simulink model "sampleModel180"  (R2021b)
settings: Solver=VariableStepAuto  StartTime=0.0  StopTime=10.0  RelTol=1e-3
undefined symbols (not defined in the file or in its folder): DiscIntNeverNeededParam, Newton, Raphson
libraries: simulink x11, slpidlib x4
settings Model: Creator=user  LastModifiedBy=user

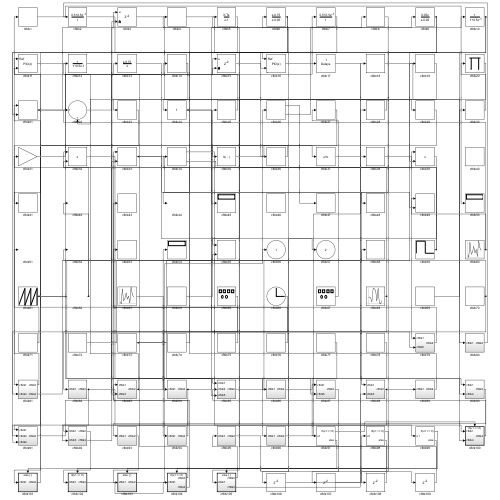
[thumbnail: Simulink's stored preview of the top-level diagram]
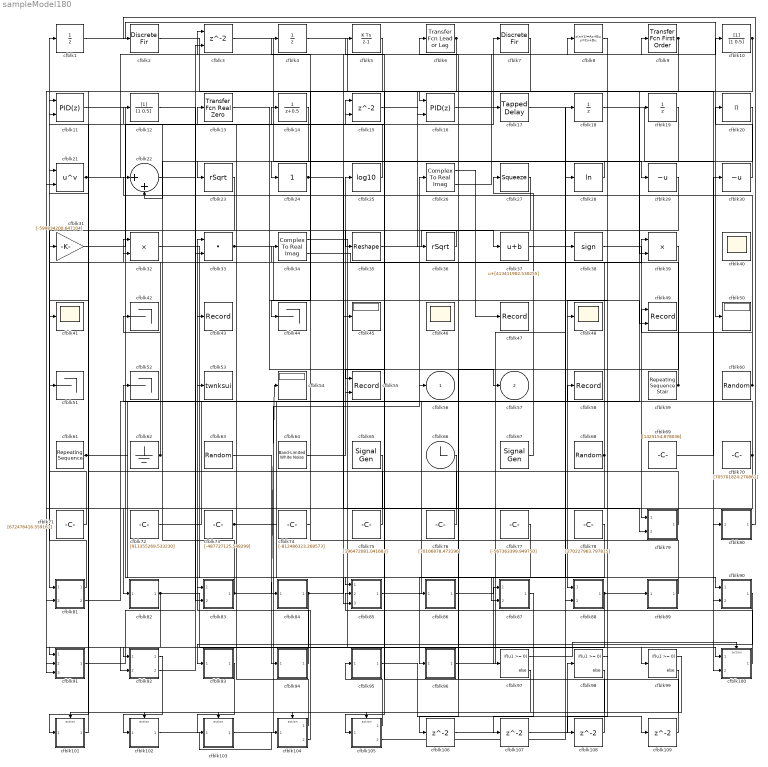
== system sampleModel180 ==
  cfblk{1,4,18..19} (4 alike) : UnitDelay  HasFrameUpgradeWarning=on
  cfblk10 : DiscreteFilter  SampleTime=1
  cfblk100 : Subsystem  TreatAsAtomicUnit=on
  cfblk101 : Subsystem  TreatAsAtomicUnit=on
  cfblk102 : Subsystem  TreatAsAtomicUnit=on
  cfblk103 : Subsystem  TreatAsAtomicUnit=on
  cfblk104 : Subsystem  TreatAsAtomicUnit=on
  cfblk105 : Subsystem  TreatAsAtomicUnit=on
  cfblk{106..109} (4 alike) : Delay  SampleTime=1
  cfblk11 : slpidlib/PID Controller (2DOF)  Controller=PID  Form=Parallel  TimeDomain=Discrete-time  UseExternalTs=off  SampleTime=1  IntegratorMethod=Forward Euler  FilterMethod=Forward Euler  ControllerParametersSource=internal  P=1  I=1  D=0  UseFilter=on  N=100  b=1  c=1  TunerSelectOption=Transfer Function Based (PID Tuner App)  InitialConditionSource=internal  InitialConditionForIntegrator=0  InitialConditionForFilter=0  DifferentiatorICPrevScaledInput=0  ExternalReset=none  TrackingMode=off  Kt=1  LimitOutput=off  SatLimitsSource=internal  UpperSaturationLimit=inf  LowerSaturationLimit=-inf  LinearizeAsGain=off  AntiWindupMode=none  Kb=1  POutMin=[]  POutMax=[]  IOutMin=[]  IOutMax=[]  DOutMin=[]  DOutMax=[]  NOutMin=[]  NOutMax=[]  bOutMin=[]  bOutMax=[]  cOutMin=[]  cOutMax=[]  SumOutMin=[]  SumOutMax=[]  SaturationOutMin=[]  SaturationOutMax=[]  PParamMin=[]  PParamMax=[]  IParamMin=[]  IParamMax=[]  DParamMin=[]  DParamMax=[]  NParamMin=[]  NParamMax=[]  bParamMin=[]  bParamMax=[]  cParamMin=[]  cParamMax=[]  KbParamMin=[]  KbParamMax=[]  KtParamMin=[]  KtParamMax=[]  KbOutMin=[]  KbOutMax=[]  KtOutMin=[]  KtOutMax=[]  IntegratorOutMin=[]  IntegratorOutMax=[]  FilterOutMin=[]  FilterOutMax=[]  SumI1OutMin=[]  SumI1OutMax=[]  SumI2OutMin=[]  SumI2OutMax=[]  SumI3OutMin=[]  SumI3OutMax=[]  SumI4OutMin=[]  SumI4OutMax=[]  SumDOutMin=[]  SumDOutMax=[]  Sum1OutMin=[]  Sum1OutMax=[]  Sum2OutMin=[]  Sum2OutMax=[]  Sum3OutMin=[]  Sum3OutMax=[]  DifferentiatorOutMin=[]  DifferentiatorOutMax=[]  FilterDiffOutCoefMin=[]  FilterDiffOutCoefMax=[]  ReciprocalOutMin=[]  ReciprocalOutMax=[]  SumDenOutMin=[]  SumDenOutMax=[]  SumNumOutMin=[]  SumNumOutMax=[]  DivideOutMin=[]  DivideOutMax=[]  UdiffTsProdOutMin=[]  UdiffTsProdOutMax=[]  NTsProdOutMin=[]  NTsProdOutMax=[]  UintegralTsProdOutMin=[]  UintegralTsProdOutMax=[]  UngainTsProdOutMin=[]  UngainTsProdOutMax=[]  IntegratorContinuousStateAttributes=''  IntegratorStateMustResolveToSignalObject=off  IntegratorRTWStateStorageClass=Auto  FilterContinuousStateAttributes=''  FilterStateMustResolveToSignalObject=off  FilterRTWStateStorageClass=Auto  ParallelPVariant=InternalParameters  IdealPVariant=Disabled  IVariant=InternalParameters  DVariant=InternalParameters  bVariant=InternalParameters  cVariant=InternalParameters  IntegratorVariant=Discrete  SatVariant=Disabled  AWVariant=Passthrough  PCopyVariant=Disabled  TRVariant=Disabled  FdbkBlocksVariant=Forward  IdealPFdbkVariant=Disabled  SatFdbkVariant=Disabled  DerivativeFilterVariant=ForwardEulerFilter  NVariant=InternalParameters  NCopyVariant=Disabled  FilterICVariant=InternalICsFilter  IntegratorICVariant=InternalICs  ExternalResetVariant=Disabled  TRSumVariant=Passthrough  SumFdbkVariant=Disabled  SumVariant=Sum_PID  TsampFilterVariant=InternalTs  TsampNgainVariant=Passthrough  TsampIntegralVariant=Passthrough  ExternalSaturationOutDataTypeStr=Inherit: Same as second input
      settings: SourceProductBaseCode=SL
  cfblk12 : DiscreteFilter  SampleTime=1
  cfblk13 : simulink/Discrete/Transfer Fcn Real Zero  ZeroZ=0.75  ICPrevInput=0.0  DoSatur=off
      settings: SourceProductBaseCode=SL
  cfblk14 : DiscreteTransferFcn  SampleTime=1
  cfblk15 : Delay  ShowEnablePort=on  SampleTime=1
      settings: InputPortMap=u0,e6
  cfblk16 : slpidlib/PID Controller (2DOF)  Controller=PID  Form=Parallel  TimeDomain=Discrete-time  UseExternalTs=off  SampleTime=1  IntegratorMethod=Forward Euler  FilterMethod=Forward Euler  ControllerParametersSource=internal  P=1  I=1  D=0  UseFilter=on  N=100  b=1  c=1  TunerSelectOption=Transfer Function Based (PID Tuner App)  InitialConditionSource=internal  InitialConditionForIntegrator=0  InitialConditionForFilter=0  DifferentiatorICPrevScaledInput=0  ExternalReset=none  TrackingMode=off  Kt=1  LimitOutput=off  SatLimitsSource=internal  UpperSaturationLimit=inf  LowerSaturationLimit=-inf  LinearizeAsGain=off  AntiWindupMode=none  Kb=1  POutMin=[]  POutMax=[]  IOutMin=[]  IOutMax=[]  DOutMin=[]  DOutMax=[]  NOutMin=[]  NOutMax=[]  bOutMin=[]  bOutMax=[]  cOutMin=[]  cOutMax=[]  SumOutMin=[]  SumOutMax=[]  SaturationOutMin=[]  SaturationOutMax=[]  PParamMin=[]  PParamMax=[]  IParamMin=[]  IParamMax=[]  DParamMin=[]  DParamMax=[]  NParamMin=[]  NParamMax=[]  bParamMin=[]  bParamMax=[]  cParamMin=[]  cParamMax=[]  KbParamMin=[]  KbParamMax=[]  KtParamMin=[]  KtParamMax=[]  KbOutMin=[]  KbOutMax=[]  KtOutMin=[]  KtOutMax=[]  IntegratorOutMin=[]  IntegratorOutMax=[]  FilterOutMin=[]  FilterOutMax=[]  SumI1OutMin=[]  SumI1OutMax=[]  SumI2OutMin=[]  SumI2OutMax=[]  SumI3OutMin=[]  SumI3OutMax=[]  SumI4OutMin=[]  SumI4OutMax=[]  SumDOutMin=[]  SumDOutMax=[]  Sum1OutMin=[]  Sum1OutMax=[]  Sum2OutMin=[]  Sum2OutMax=[]  Sum3OutMin=[]  Sum3OutMax=[]  DifferentiatorOutMin=[]  DifferentiatorOutMax=[]  FilterDiffOutCoefMin=[]  FilterDiffOutCoefMax=[]  ReciprocalOutMin=[]  ReciprocalOutMax=[]  SumDenOutMin=[]  SumDenOutMax=[]  SumNumOutMin=[]  SumNumOutMax=[]  DivideOutMin=[]  DivideOutMax=[]  UdiffTsProdOutMin=[]  UdiffTsProdOutMax=[]  NTsProdOutMin=[]  NTsProdOutMax=[]  UintegralTsProdOutMin=[]  UintegralTsProdOutMax=[]  UngainTsProdOutMin=[]  UngainTsProdOutMax=[]  IntegratorContinuousStateAttributes=''  IntegratorStateMustResolveToSignalObject=off  IntegratorRTWStateStorageClass=Auto  FilterContinuousStateAttributes=''  FilterStateMustResolveToSignalObject=off  FilterRTWStateStorageClass=Auto  ParallelPVariant=InternalParameters  IdealPVariant=Disabled  IVariant=InternalParameters  DVariant=InternalParameters  bVariant=InternalParameters  cVariant=InternalParameters  IntegratorVariant=Discrete  SatVariant=Disabled  AWVariant=Passthrough  PCopyVariant=Disabled  TRVariant=Disabled  FdbkBlocksVariant=Forward  IdealPFdbkVariant=Disabled  SatFdbkVariant=Disabled  DerivativeFilterVariant=ForwardEulerFilter  NVariant=InternalParameters  NCopyVariant=Disabled  FilterICVariant=InternalICsFilter  IntegratorICVariant=InternalICs  ExternalResetVariant=Disabled  TRSumVariant=Passthrough  SumFdbkVariant=Disabled  SumVariant=Sum_PID  TsampFilterVariant=InternalTs  TsampNgainVariant=Passthrough  TsampIntegralVariant=Passthrough  ExternalSaturationOutDataTypeStr=Inherit: Same as second input
      settings: SourceProductBaseCode=SL
  cfblk17 : simulink/Discrete/Tapped Delay  vinit=0.0  samptime=-1  NumDelays=1  DelayOrder=Oldest  includeCurrent=off
  cfblk2 : DiscreteFir  SampleTime=1
  cfblk20 : Product  Inputs=*
  cfblk21 : Math  Operator=pow  SaturateOnIntegerOverflow=on
  cfblk22 : Sum  Inputs=|++
  cfblk23 : Sqrt  Operator=rSqrt  AlgorithmType=Newton-Raphson  SaturateOnIntegerOverflow=on
  cfblk24 : simulink/Math Operations/Slider Gain  gain=1  low=0  high=2
  cfblk25 : Math  Operator=log10  SaturateOnIntegerOverflow=on
  cfblk26 : ComplexToRealImag
  cfblk27 : Squeeze
  cfblk28 : Math  Operator=log  SaturateOnIntegerOverflow=on
  cfblk29 : UnaryMinus
  cfblk3 : Delay  ShowEnablePort=on  SampleTime=1
      settings: InputPortMap=u0,e6
  cfblk30 : UnaryMinus
  cfblk31 : Gain  Gain=[-599834200.647104]
  cfblk32 : Product
  cfblk33 : DotProduct  InputSameDT=on  OutDataTypeStr=Inherit: Inherit via internal rule
  cfblk34 : ComplexToRealImag
  cfblk35 : Reshape
  cfblk36 : Sqrt  Operator=rSqrt  AlgorithmType=Newton-Raphson  SaturateOnIntegerOverflow=on
  cfblk37 : Bias  Bias=[413411902.530255]
  cfblk38 : Signum
  cfblk39 : Product
  cfblk{40..41,46,48} (4 alike) : Scope
      cfblk40 settings: Floating=on
      cfblk46 settings: Floating=on
  cfblk{42,44,51..52} (4 alike) : Terminator
  cfblk43 : Record  FileSettingsInternal="{\"entries\":[{\"content\":{\"excelSettings\":{\"content\":{},\"type\":\"Streamout.ExcelSettings\"}},\"type\":\"Streamout.FileSettingStorage\",\"uuid\":\"86445610-928e-4e35-9d69-0b2c780a0add\"}],\"packageUris\":[\"http://schema.mathworks.com/mf0/streamout_blocks/R2020a\"],\"version\":\"1.0\"}"  SignalsInternal="{\"entries\":[{\"content\":{\"signals\":[{\"content\":{\"blockPath\":[\"sampleModel180/cfblk43\"],\"channel\":[],\"dimensions\":[1],\"domain\":\"sampleModel180/cfblk43\",\"lineColor\":\"#4dbeee\",\"plots\":[1],\"port\":1,\"sid\":[\"\"],\"signalID\":6746,\"signalName\":\"cfblk79\"},\"type\":\"RecordBlkView.Signal\",\"uuid\":\"ec482149-7623-4eb4-899c-afc25818783d\"}]},\"type\":\"RecordBlkView.InputSignals\",\"uuid\":\"a47f1734-a9d2-497d-b596-b6906e889272\"}],\"packageUris\":[\"http://schema.mathworks.com/mf0/streamout_blocks/R2020a\"],\"version\":\"1.0\"}"  VisualizationBindings="{\"sparklinesplugin\":{\"info\":[{\"bindingParametersList\":[],\"subplotID\":1}]}}"
  cfblk45 : Display
  cfblk47 : Record  FileSettingsInternal="{\"entries\":[{\"content\":{\"excelSettings\":{\"content\":{},\"type\":\"Streamout.ExcelSettings\"}},\"type\":\"Streamout.FileSettingStorage\",\"uuid\":\"e1298681-f42b-4617-9df3-3c8d902f72c9\"}],\"packageUris\":[\"http://schema.mathworks.com/mf0/streamout_blocks/R2020a\"],\"version\":\"1.0\"}"  SignalsInternal="{\"entries\":[{\"content\":{\"signals\":[{\"content\":{\"blockPath\":[\"sampleModel180/cfblk47\"],\"channel\":[],\"dimensions\":[1],\"domain\":\"sampleModel180/cfblk47\",\"lineColor\":\"#a2142f\",\"plots\":[1],\"port\":1,\"sid\":[\"\"],\"signalID\":6750,\"signalName\":\"cfblk26:1\"},\"type\":\"RecordBlkView.Signal\",\"uuid\":\"9f111c3f-576d-47fa-9d33-bb703aee1316\"}]},\"type\":\"RecordBlkView.InputSignals\",\"uuid\":\"73cee130-5659-46ca-9b54-9eadd692a438\"}],\"packageUris\":[\"http://schema.mathworks.com/mf0/streamout_blocks/R2020a\"],\"version\":\"1.0\"}"  VisualizationBindings="{\"sparklinesplugin\":{\"info\":[{\"bindingParametersList\":[],\"subplotID\":1}]}}"
  cfblk49 : Record  FileSettingsInternal="{\"entries\":[{\"content\":{\"excelSettings\":{\"content\":{},\"type\":\"Streamout.ExcelSettings\"}},\"type\":\"Streamout.FileSettingStorage\",\"uuid\":\"1f60f6e5-b911-44b5-b854-fc3e9ae4dd78\"}],\"packageUris\":[\"http://schema.mathworks.com/mf0/streamout_blocks/R2020a\"],\"version\":\"1.0\"}"  Layout=[1 1]  SignalsInternal="{\"entries\":[{\"content\":{\"signals\":[{\"content\":{\"blockPath\":[\"sampleModel180/cfblk49\"],\"channel\":[],\"dimensions\":[1],\"domain\":\"sampleModel180/cfblk49\",\"lineColor\":\"#a2142f\",\"plots\":[1],\"port\":1,\"sid\":[\"\"],\"signalID\":6754,\"signalName\":\"cfblk60\"},\"type\":\"RecordBlkView.Signal\",\"uuid\":\"31debbde-8abb-4355-a209-1ad38695556c\"},{\"content\":{\"blockPath\":[\"sampleModel180/cfblk49\"],\"channel\":[],\"dimensions\":[1],\"domain\":\"sampleModel180/cfblk49\",\"lineColor\":\"#139fff\",\"plots\":[1],\"port\":2,\"sid\":[\"\"],\"signalID\":6758,\"signalName\":\"cfblk33\"},\"type\":\"RecordBlkView.Signal\",\"uuid\":\"d752f508-f027-4e5d-b6d4-7f1136115733\"}]},\"type\":\"RecordBlkView.InputSignals\",\"uuid\":\"6e205f7c-5895-4b43-953f-c0e2bfe62826\"}],\"packageUris\":[\"http://schema.mathworks.com/mf0/streamout_blocks/R2020a\"],\"version\":\"1.0\"}"  VisualizationBindings="{\"xyplotplugin\":{\"info\":[{\"series\":[{\"bindingParametersList\":[{\"parameter\":\"X-Axis\",\"signalID\":6754,\"signalName\":\"cfblk60\"},{\"parameter\":\"Y-Axis\",\"signalID\":6758,\"signalName\":\"cfblk33\"}],\"seriesID\":2376}],\"subplotID\":1}]}}"  CompatibilityTag=XY
  cfblk5 : DiscreteIntegrator  ICPrevOutput=DiscIntNeverNeededParam  ICPrevScaledInput=DiscIntNeverNeededParam
  cfblk50 : Display
  cfblk53 : ToWorkspace  VariableName=twnksui  SaveFormat=Timeseries  SampleTime=-1
  cfblk54 : Display
  cfblk55 : Record  FileSettingsInternal="{\"entries\":[{\"content\":{\"excelSettings\":{\"content\":{},\"type\":\"Streamout.ExcelSettings\"}},\"type\":\"Streamout.FileSettingStorage\",\"uuid\":\"12a34ce2-1638-4df7-a144-cdb538d8a942\"}],\"packageUris\":[\"http://schema.mathworks.com/mf0/streamout_blocks/R2020a\"],\"version\":\"1.0\"}"  Layout=[1 1]  SignalsInternal="{\"entries\":[{\"content\":{\"signals\":[{\"content\":{\"blockPath\":[\"sampleModel180/cfblk55\"],\"channel\":[],\"dimensions\":[1],\"domain\":\"sampleModel180/cfblk55\",\"lineColor\":\"#a2142f\",\"plots\":[1],\"port\":1,\"sid\":[\"\"],\"signalID\":6762,\"signalName\":\"cfblk19\"},\"type\":\"RecordBlkView.Signal\",\"uuid\":\"c6582ab4-e272-4f30-9ee4-33b16e3ab7cf\"},{\"content\":{\"blockPath\":[\"sampleModel180/cfblk55\"],\"channel\":[],\"dimensions\":[1],\"domain\":\"sampleModel180/cfblk55\",\"lineColor\":\"#139fff\",\"plots\":[1],\"port\":2,\"sid\":[\"\"],\"signalID\":6766,\"signalName\":\"cfblk64\"},\"type\":\"RecordBlkView.Signal\",\"uuid\":\"59037f3a-43fc-4b4b-b1ee-851af1b0e0dd\"}]},\"type\":\"RecordBlkView.InputSignals\",\"uuid\":\"311858ce-66bd-4406-93c2-197a3cee1eee\"}],\"packageUris\":[\"http://schema.mathworks.com/mf0/streamout_blocks/R2020a\"],\"version\":\"1.0\"}"  VisualizationBindings="{\"xyplotplugin\":{\"info\":[{\"series\":[{\"bindingParametersList\":[{\"parameter\":\"X-Axis\",\"signalID\":6762,\"signalName\":\"cfblk19\"},{\"parameter\":\"Y-Axis\",\"signalID\":6766,\"signalName\":\"cfblk64\"}],\"seriesID\":41445}],\"subplotID\":1}]}}"  CompatibilityTag=XY
  cfblk58 : Record  FileSettingsInternal="{\"entries\":[{\"content\":{\"excelSettings\":{\"content\":{},\"type\":\"Streamout.ExcelSettings\"}},\"type\":\"Streamout.FileSettingStorage\",\"uuid\":\"8464cd75-87e0-42e4-b570-b7ba8dcc5bb1\"}],\"packageUris\":[\"http://schema.mathworks.com/mf0/streamout_blocks/R2020a\"],\"version\":\"1.0\"}"  SignalsInternal="{\"entries\":[{\"content\":{\"signals\":[{\"content\":{\"blockPath\":[\"sampleModel180/cfblk58\"],\"channel\":[],\"dimensions\":[1],\"domain\":\"sampleModel180/cfblk58\",\"lineColor\":\"#ff13a6\",\"plots\":[1],\"port\":1,\"sid\":[\"\"],\"signalID\":6770,\"signalName\":\"cfblk85\"},\"type\":\"RecordBlkView.Signal\",\"uuid\":\"29ee1141-0291-4ef1-9b75-827cb369f832\"}]},\"type\":\"RecordBlkView.InputSignals\",\"uuid\":\"9077ce9c-33ad-41e5-ad34-2c1f7967bf27\"}],\"packageUris\":[\"http://schema.mathworks.com/mf0/streamout_blocks/R2020a\"],\"version\":\"1.0\"}"  VisualizationBindings="{\"sparklinesplugin\":{\"info\":[{\"bindingParametersList\":[],\"subplotID\":1}]}}"
  cfblk59 : simulink/Sources/Repeating Sequence Stair  OutValues=[766336489.541645, 669322313.882846]  tsamp=-1  OutMin=[]  OutMax=[]  OutDataTypeStr=double  OutputDataTypeScalingMode=double  OutDataType=fixdt(0,8)  ConRadixGroup=Best Precision: Vector-wise  OutScaling=2^-12
  cfblk6 : simulink/Discrete/Transfer Fcn Lead or Lag  PoleZ=0.95  ZeroZ=0.75  ICPrevOutput=0.0  ICPrevInput=0.0  DoSatur=off
      settings: SourceProductBaseCode=SL
  cfblk60 : UniformRandomNumber  Minimum=[-5912958699.125717]  Maximum=[7739222347.469520]  Seed=[40590671.000000]  SampleTime=0.1
  cfblk61 : simulink/Sources/Repeating Sequence  rep_seq_t=[0 2]  rep_seq_y=[-660048765.105391, -46648414.470810]
  cfblk62 : Ground
  cfblk63 : UniformRandomNumber  Minimum=[-2646210687.817862]  Maximum=[3798625207.117166]  Seed=[15842271.000000]  SampleTime=0.1
  cfblk64 : simulink/Sources/Band-Limited White Noise  Cov=[4480573628.038885]  Ts=0.1  seed=[6249292123.000000]
  cfblk65 : SignalGenerator  Amplitude=[464475926.182295]  Units=rad/sec
  cfblk66 : Clock
  cfblk67 : SignalGenerator  WaveForm=square  Amplitude=[-424263037.736154]
  cfblk68 : RandomNumber  Mean=[-24659.259626]  Variance=[97657.847549]  Seed=[139015399.000000]  SampleTime=0.1
  cfblk69 : Constant  Value=[1425154.878036]  SampleTime=1
  cfblk7 : DiscreteFir  SampleTime=1
  cfblk70 : Constant  Value=[705701824.270861]  SampleTime=1
  cfblk71 : Constant  Value=[672476416.559161]  SampleTime=1
  cfblk72 : Constant  Value=[911355269.533230]  SampleTime=1
  cfblk73 : Constant  Value=[-487727125.548299]  SampleTime=1
  cfblk74 : Constant  Value=[-812486323.268573]  SampleTime=1
  cfblk75 : Constant  Value=[196472081.041683]  SampleTime=1
  cfblk76 : Constant  Value=[70106878.473196]  SampleTime=1
  cfblk77 : Constant  Value=[-567363399.949750]  SampleTime=1
  cfblk78 : Constant  Value=[270227963.797815]  SampleTime=1
  cfblk79 : Subsystem
  cfblk8 : DiscreteStateSpace
  cfblk80 : Subsystem
  cfblk81 : Subsystem
  cfblk82 : Subsystem
  cfblk83 : Subsystem
  cfblk84 : Subsystem
  cfblk85 : Subsystem
  cfblk86 : Subsystem
  cfblk87 : Subsystem
  cfblk88 : Subsystem
  cfblk89 : Subsystem
  cfblk9 : simulink/Discrete/Transfer Fcn First Order  PoleZ=0.95  ICPrevOutput=0.0  DoSatur=off
  cfblk90 : Subsystem
  cfblk91 : Subsystem
  cfblk92 : Subsystem
  cfblk93 : Subsystem
  cfblk94 : Subsystem
  cfblk95 : Subsystem
  cfblk96 : Subsystem
  cfblk97 : If  IfExpression=u1 >= 0  SampleTime=1
  cfblk98 : If  IfExpression=u1 >= 0  SampleTime=1
  cfblk99 : If  IfExpression=u1 >= 0  SampleTime=1
  cfblk56 : Outport
  cfblk57 : Outport  Port=2
  wires:
  cfblk72/1 -> cfblk25/1
  cfblk14/1 -> cfblk23/1
  cfblk26/1 -> cfblk47/1
  cfblk9/1 -> cfblk44/1, cfblk16/2
  cfblk1/1 -> cfblk50/1
  cfblk103/1(cfblk2) -> cfblk26/1
  cfblk37/1 -> cfblk38/1
  cfblk23/1 -> cfblk81/1(cfblk1)
  cfblk3/1 -> cfblk29/1
  cfblk34/1 -> cfblk100/1(cfblk1)
  cfblk35/1 -> cfblk37/1
  cfblk71/1 -> cfblk1/1
  cfblk104/1(cfblk2) -> cfblk13/1
  cfblk66/1 -> cfblk81/2(cfblk3)
  cfblk101/1(cfblk2) -> cfblk31/1
  cfblk88/1(cfblk2) -> cfblk89/1(cfblk1), cfblk92/1(cfblk1)
  cfblk105/1(cfblk2) -> cfblk95/1(cfblk1)
  cfblk33/1 -> cfblk88/1(cfblk1), cfblk49/2
  cfblk25/1 -> cfblk11/1
  cfblk11/1 -> cfblk85/1(cfblk1)
  cfblk16/1 -> cfblk7/1
  cfblk36/1 -> cfblk35/1
  cfblk12/1 -> cfblk90/1(cfblk1)
  cfblk19/1 -> cfblk55/1
  cfblk31/1 -> cfblk15/1
  cfblk18/1 -> cfblk100/2(cfblk4)
  cfblk74/1 -> cfblk4/1
  cfblk22/1 -> cfblk9/1
  cfblk24/1 -> cfblk45/1, cfblk79/2(cfblk5)
  cfblk21/1 -> cfblk14/1, cfblk3/1
  cfblk80/1(cfblk2) -> cfblk2/1
  cfblk34/2 -> cfblk39/1
  cfblk10/1 -> cfblk48/1, cfblk39/2
  cfblk96/1(cfblk2) -> cfblk18/1
  cfblk78/1 -> cfblk97/1
  cfblk81/1(cfblk2) -> cfblk51/1
  cfblk89/1(cfblk2) -> cfblk34/1
  cfblk82/1(cfblk2) -> cfblk99/1, cfblk92/2(cfblk3)
  cfblk85/1(cfblk2) -> cfblk58/1
  cfblk86/1(cfblk2) -> cfblk87/1(cfblk1)
  cfblk61/1 -> cfblk96/1(cfblk1), cfblk3/2
  cfblk94/1(cfblk2) -> cfblk33/1
  cfblk6/1 -> cfblk105/1(cfblk1), cfblk91/3(cfblk4)
  cfblk69/1 -> cfblk30/1
  cfblk73/1 -> cfblk19/1, cfblk85/3(cfblk5)
  cfblk102/1(cfblk2) -> cfblk104/1(cfblk1)
  cfblk105/2(cfblk4) -> cfblk28/1
  cfblk60/1 -> cfblk22/1, cfblk49/1
  cfblk29/1 -> cfblk101/1(cfblk1)
  cfblk70/1 -> cfblk52/1, cfblk84/1(cfblk1)
  cfblk68/1 -> cfblk32/1, cfblk83/2(cfblk3)
  cfblk30/1 -> cfblk20/1
  cfblk32/1 -> cfblk87/2(cfblk5)
  cfblk38/1 -> cfblk79/1(cfblk1)
  cfblk59/1 -> cfblk12/1, cfblk15/2
  cfblk93/1(cfblk2) -> cfblk103/1(cfblk1)
  cfblk65/1 -> cfblk82/1(cfblk1)
  cfblk4/1 -> cfblk80/1(cfblk1)
  cfblk100/1(cfblk2) -> cfblk85/2(cfblk4)
  cfblk90/1(cfblk2) -> cfblk93/1(cfblk1)
  cfblk92/1(cfblk2) -> cfblk102/1(cfblk1)
  cfblk81/2(cfblk4) -> cfblk56/1
  cfblk79/1(cfblk2) -> cfblk43/1
  cfblk77/1 -> cfblk86/1(cfblk1)
  cfblk5/1 -> cfblk91/1(cfblk1)
  cfblk84/1(cfblk2) -> cfblk91/2(cfblk3), cfblk10/1
  cfblk91/1(cfblk2) -> cfblk33/2
  cfblk104/2(cfblk4) -> cfblk83/1(cfblk1)
  cfblk27/1 -> cfblk41/1
  cfblk83/1(cfblk2) -> cfblk54/1, cfblk32/2
  cfblk20/1 -> cfblk22/2
  cfblk63/1 -> cfblk94/1(cfblk1)
  cfblk17/1 -> cfblk90/2(cfblk4)
  cfblk28/1 -> cfblk24/1
  cfblk15/1 -> cfblk36/1
  cfblk2/1 -> cfblk16/1
  cfblk76/1 -> cfblk53/1
  cfblk92/2(cfblk4) -> cfblk17/1
  cfblk67/1 -> cfblk27/1
  cfblk75/1 -> cfblk21/1
  cfblk64/1 -> cfblk55/2
  cfblk7/1 -> cfblk21/2
  cfblk62/1 -> cfblk42/1, cfblk11/2
  cfblk26/2 -> cfblk8/1
  cfblk13/1 -> cfblk57/1
  cfblk97/1 -> cfblk100/Action
  cfblk97/2 -> cfblk101/Action
  cfblk98/1 -> cfblk102/Action
  cfblk98/2 -> cfblk103/Action
  cfblk99/1 -> cfblk104/Action
  cfblk99/2 -> cfblk105/Action
  cfblk39/1 -> cfblk106/1
  cfblk106/1 -> cfblk88/2(cfblk3)
  cfblk87/1(cfblk2) -> cfblk107/1
  cfblk107/1 -> cfblk98/1
  cfblk8/1 -> cfblk108/1
  cfblk108/1 -> cfblk5/1
  cfblk95/1(cfblk2) -> cfblk109/1
  cfblk109/1 -> cfblk6/1

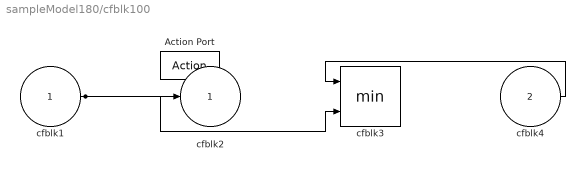
== system sampleModel180/cfblk100 ==
  cfblk1 : Inport
  cfblk4 : Inport  Port=2
  Action Port : ActionPort  ActionPortLabel=if(u1 >= 0)
  cfblk3 : MinMax  Inputs=2
  cfblk2 : Outport
  wires:
  cfblk4/1 -> cfblk3/1
  cfblk1/1 -> cfblk2/1, cfblk3/2

== system sampleModel180/cfblk101 ==
  cfblk1 : Inport
  Action Port : ActionPort  ActionPortLabel=else
  cfblk3 : slpidlib/PID Controller (2DOF)  Controller=PID  Form=Parallel  TimeDomain=Discrete-time  UseExternalTs=off  SampleTime=-1  IntegratorMethod=Forward Euler  FilterMethod=Forward Euler  ControllerParametersSource=internal  P=1  I=1  D=0  UseFilter=on  N=100  b=1  c=1  TunerSelectOption=Transfer Function Based (PID Tuner App)  InitialConditionSource=internal  InitialConditionForIntegrator=0  InitialConditionForFilter=0  DifferentiatorICPrevScaledInput=0  ExternalReset=none  TrackingMode=off  Kt=1  LimitOutput=off  SatLimitsSource=internal  UpperSaturationLimit=inf  LowerSaturationLimit=-inf  LinearizeAsGain=off  AntiWindupMode=none  Kb=1  POutMin=[]  POutMax=[]  IOutMin=[]  IOutMax=[]  DOutMin=[]  DOutMax=[]  NOutMin=[]  NOutMax=[]  bOutMin=[]  bOutMax=[]  cOutMin=[]  cOutMax=[]  SumOutMin=[]  SumOutMax=[]  SaturationOutMin=[]  SaturationOutMax=[]  PParamMin=[]  PParamMax=[]  IParamMin=[]  IParamMax=[]  DParamMin=[]  DParamMax=[]  NParamMin=[]  NParamMax=[]  bParamMin=[]  bParamMax=[]  cParamMin=[]  cParamMax=[]  KbParamMin=[]  KbParamMax=[]  KtParamMin=[]  KtParamMax=[]  KbOutMin=[]  KbOutMax=[]  KtOutMin=[]  KtOutMax=[]  IntegratorOutMin=[]  IntegratorOutMax=[]  FilterOutMin=[]  FilterOutMax=[]  SumI1OutMin=[]  SumI1OutMax=[]  SumI2OutMin=[]  SumI2OutMax=[]  SumI3OutMin=[]  SumI3OutMax=[]  SumI4OutMin=[]  SumI4OutMax=[]  SumDOutMin=[]  SumDOutMax=[]  Sum1OutMin=[]  Sum1OutMax=[]  Sum2OutMin=[]  Sum2OutMax=[]  Sum3OutMin=[]  Sum3OutMax=[]  DifferentiatorOutMin=[]  DifferentiatorOutMax=[]  FilterDiffOutCoefMin=[]  FilterDiffOutCoefMax=[]  ReciprocalOutMin=[]  ReciprocalOutMax=[]  SumDenOutMin=[]  SumDenOutMax=[]  SumNumOutMin=[]  SumNumOutMax=[]  DivideOutMin=[]  DivideOutMax=[]  UdiffTsProdOutMin=[]  UdiffTsProdOutMax=[]  NTsProdOutMin=[]  NTsProdOutMax=[]  UintegralTsProdOutMin=[]  UintegralTsProdOutMax=[]  UngainTsProdOutMin=[]  UngainTsProdOutMax=[]  IntegratorContinuousStateAttributes=''  IntegratorStateMustResolveToSignalObject=off  IntegratorRTWStateStorageClass=Auto  FilterContinuousStateAttributes=''  FilterStateMustResolveToSignalObject=off  FilterRTWStateStorageClass=Auto  ParallelPVariant=InternalParameters  IdealPVariant=Disabled  IVariant=InternalParameters  DVariant=InternalParameters  bVariant=InternalParameters  cVariant=InternalParameters  IntegratorVariant=Discrete  SatVariant=Disabled  AWVariant=Passthrough  PCopyVariant=Disabled  TRVariant=Disabled  FdbkBlocksVariant=Forward  IdealPFdbkVariant=Disabled  SatFdbkVariant=Disabled  DerivativeFilterVariant=ForwardEulerFilter  NVariant=InternalParameters  NCopyVariant=Disabled  FilterICVariant=InternalICsFilter  IntegratorICVariant=InternalICs  ExternalResetVariant=Disabled  TRSumVariant=Passthrough  SumFdbkVariant=Disabled  SumVariant=Sum_PID  TsampFilterVariant=InternalTs  TsampNgainVariant=Passthrough  TsampIntegralVariant=Passthrough  ExternalSaturationOutDataTypeStr=Inherit: Same as second input
      settings: SourceProductBaseCode=SL
  cfblk2 : Outport
  wires:
  cfblk1/1 -> cfblk2/1, cfblk3/1, cfblk3/2

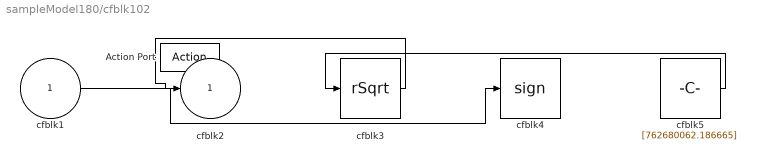
== system sampleModel180/cfblk102 ==
  cfblk1 : Inport
  Action Port : ActionPort  ActionPortLabel=if(u1 >= 0)
  cfblk3 : Sqrt  Operator=rSqrt  AlgorithmType=Newton-Raphson  SaturateOnIntegerOverflow=on
  cfblk4 : Signum
  cfblk5 : Constant  Value=[762680062.186665]  SampleTime=1
  cfblk2 : Outport
  wires:
  cfblk1/1 -> cfblk4/1
  cfblk3/1 -> cfblk2/1
  cfblk5/1 -> cfblk3/1

== system sampleModel180/cfblk103 ==
  cfblk1 : Inport
  Action Port : ActionPort  ActionPortLabel=else
  cfblk3 : Delay
  cfblk2 : Outport
  wires:
  cfblk1/1 -> cfblk3/1
  cfblk3/1 -> cfblk2/1

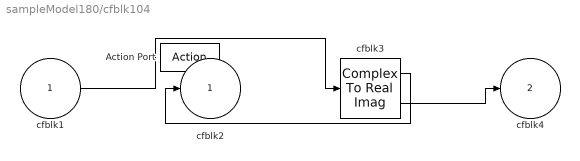
== system sampleModel180/cfblk104 ==
  cfblk1 : Inport
  Action Port : ActionPort  ActionPortLabel=if(u1 >= 0)
  cfblk3 : ComplexToRealImag
  cfblk2 : Outport
  cfblk4 : Outport  Port=2
  wires:
  cfblk3/1 -> cfblk2/1
  cfblk1/1 -> cfblk3/1
  cfblk3/2 -> cfblk4/1

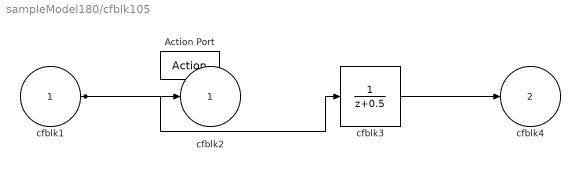
== system sampleModel180/cfblk105 ==
  cfblk1 : Inport
  Action Port : ActionPort  ActionPortLabel=else
  cfblk3 : DiscreteTransferFcn
  cfblk2 : Outport
  cfblk4 : Outport  Port=2
  wires:
  cfblk3/1 -> cfblk4/1
  cfblk1/1 -> cfblk2/1, cfblk3/1

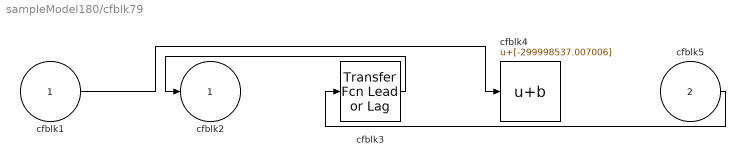
== system sampleModel180/cfblk79 ==
  cfblk1 : Inport
  cfblk5 : Inport  Port=2
  cfblk3 : simulink/Discrete/Transfer Fcn Lead or Lag  PoleZ=0.95  ZeroZ=0.75  ICPrevOutput=0.0  ICPrevInput=0.0  DoSatur=off
      settings: SourceProductBaseCode=SL
  cfblk4 : Bias  Bias=[-299998537.007006]
  cfblk2 : Outport
  wires:
  cfblk3/1 -> cfblk2/1
  cfblk5/1 -> cfblk3/1
  cfblk1/1 -> cfblk4/1

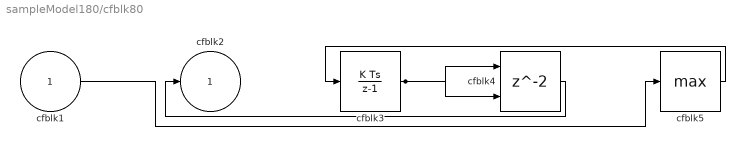
== system sampleModel180/cfblk80 ==
  cfblk1 : Inport
  cfblk3 : DiscreteIntegrator  ICPrevOutput=DiscIntNeverNeededParam  ICPrevScaledInput=DiscIntNeverNeededParam
  cfblk4 : Delay  ShowEnablePort=on  SampleTime=1
      settings: InputPortMap=u0,e6
  cfblk5 : MinMax  Function=max
  cfblk2 : Outport
  wires:
  cfblk5/1 -> cfblk3/1
  cfblk4/1 -> cfblk2/1
  cfblk3/1 -> cfblk4/1, cfblk4/2
  cfblk1/1 -> cfblk5/1

== system sampleModel180/cfblk81 ==
  cfblk1 : Inport
  cfblk3 : Inport  Port=2
  cfblk2 : Outport
  cfblk4 : Outport  Port=2
  wires:
  cfblk1/1 -> cfblk2/1
  cfblk3/1 -> cfblk4/1

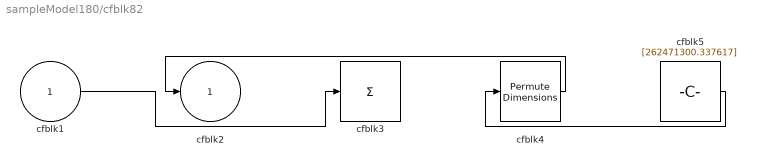
== system sampleModel180/cfblk82 ==
  cfblk1 : Inport
  cfblk3 : Sum  Inputs=+
  cfblk4 : PermuteDimensions
  cfblk5 : Constant  Value=[262471300.337617]  SampleTime=1
  cfblk2 : Outport
  wires:
  cfblk4/1 -> cfblk2/1
  cfblk5/1 -> cfblk4/1
  cfblk1/1 -> cfblk3/1

== system sampleModel180/cfblk83 ==
  cfblk1 : Inport
  cfblk3 : Inport  Port=2
  cfblk2 : Outport
  wires:
  cfblk1/1 -> cfblk2/1

== system sampleModel180/cfblk84 ==
  cfblk1 : Inport
  cfblk3 : Delay  DelayLengthSource=Input port  SampleTime=1
      settings: InputPortMap=u0,p1
  cfblk4 : Bias  Bias=[-608128811.975170]
  cfblk2 : Outport
  wires:
  cfblk4/1 -> cfblk2/1, cfblk3/1
  cfblk1/1 -> cfblk4/1, cfblk3/2

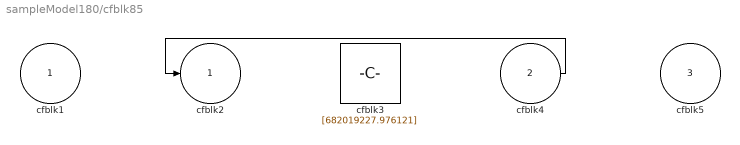
== system sampleModel180/cfblk85 ==
  cfblk1 : Inport
  cfblk4 : Inport  Port=2
  cfblk5 : Inport  Port=3
  cfblk3 : Constant  Value=[682019227.976121]  SampleTime=1
  cfblk2 : Outport
  wires:
  cfblk4/1 -> cfblk2/1

== system sampleModel180/cfblk86 ==
  cfblk1 : Inport
  cfblk3 : DiscreteFilter  SampleTime=1
  cfblk4 : slpidlib/PID Controller (2DOF)  Controller=PID  Form=Parallel  TimeDomain=Discrete-time  UseExternalTs=off  SampleTime=1  IntegratorMethod=Forward Euler  FilterMethod=Forward Euler  ControllerParametersSource=internal  P=1  I=1  D=0  UseFilter=on  N=100  b=1  c=1  TunerSelectOption=Transfer Function Based (PID Tuner App)  InitialConditionSource=internal  InitialConditionForIntegrator=0  InitialConditionForFilter=0  DifferentiatorICPrevScaledInput=0  ExternalReset=none  TrackingMode=off  Kt=1  LimitOutput=off  SatLimitsSource=internal  UpperSaturationLimit=inf  LowerSaturationLimit=-inf  LinearizeAsGain=off  AntiWindupMode=none  Kb=1  POutMin=[]  POutMax=[]  IOutMin=[]  IOutMax=[]  DOutMin=[]  DOutMax=[]  NOutMin=[]  NOutMax=[]  bOutMin=[]  bOutMax=[]  cOutMin=[]  cOutMax=[]  SumOutMin=[]  SumOutMax=[]  SaturationOutMin=[]  SaturationOutMax=[]  PParamMin=[]  PParamMax=[]  IParamMin=[]  IParamMax=[]  DParamMin=[]  DParamMax=[]  NParamMin=[]  NParamMax=[]  bParamMin=[]  bParamMax=[]  cParamMin=[]  cParamMax=[]  KbParamMin=[]  KbParamMax=[]  KtParamMin=[]  KtParamMax=[]  KbOutMin=[]  KbOutMax=[]  KtOutMin=[]  KtOutMax=[]  IntegratorOutMin=[]  IntegratorOutMax=[]  FilterOutMin=[]  FilterOutMax=[]  SumI1OutMin=[]  SumI1OutMax=[]  SumI2OutMin=[]  SumI2OutMax=[]  SumI3OutMin=[]  SumI3OutMax=[]  SumI4OutMin=[]  SumI4OutMax=[]  SumDOutMin=[]  SumDOutMax=[]  Sum1OutMin=[]  Sum1OutMax=[]  Sum2OutMin=[]  Sum2OutMax=[]  Sum3OutMin=[]  Sum3OutMax=[]  DifferentiatorOutMin=[]  DifferentiatorOutMax=[]  FilterDiffOutCoefMin=[]  FilterDiffOutCoefMax=[]  ReciprocalOutMin=[]  ReciprocalOutMax=[]  SumDenOutMin=[]  SumDenOutMax=[]  SumNumOutMin=[]  SumNumOutMax=[]  DivideOutMin=[]  DivideOutMax=[]  UdiffTsProdOutMin=[]  UdiffTsProdOutMax=[]  NTsProdOutMin=[]  NTsProdOutMax=[]  UintegralTsProdOutMin=[]  UintegralTsProdOutMax=[]  UngainTsProdOutMin=[]  UngainTsProdOutMax=[]  IntegratorContinuousStateAttributes=''  IntegratorStateMustResolveToSignalObject=off  IntegratorRTWStateStorageClass=Auto  FilterContinuousStateAttributes=''  FilterStateMustResolveToSignalObject=off  FilterRTWStateStorageClass=Auto  ParallelPVariant=InternalParameters  IdealPVariant=Disabled  IVariant=InternalParameters  DVariant=InternalParameters  bVariant=InternalParameters  cVariant=InternalParameters  IntegratorVariant=Discrete  SatVariant=Disabled  AWVariant=Passthrough  PCopyVariant=Disabled  TRVariant=Disabled  FdbkBlocksVariant=Forward  IdealPFdbkVariant=Disabled  SatFdbkVariant=Disabled  DerivativeFilterVariant=ForwardEulerFilter  NVariant=InternalParameters  NCopyVariant=Disabled  FilterICVariant=InternalICsFilter  IntegratorICVariant=InternalICs  ExternalResetVariant=Disabled  TRSumVariant=Passthrough  SumFdbkVariant=Disabled  SumVariant=Sum_PID  TsampFilterVariant=InternalTs  TsampNgainVariant=Passthrough  TsampIntegralVariant=Passthrough  ExternalSaturationOutDataTypeStr=Inherit: Same as second input
      settings: SourceProductBaseCode=SL
  cfblk5 : Constant  Value=[267636538.716776]  SampleTime=1
  cfblk2 : Outport
  wires:
  cfblk4/1 -> cfblk3/1
  cfblk5/1 -> cfblk4/1
  cfblk1/1 -> cfblk4/2
  cfblk3/1 -> cfblk2/1

== system sampleModel180/cfblk87 ==
  cfblk1 : Inport
  cfblk5 : Inport  Port=2
  cfblk3 : simulink/Discrete/Transfer Fcn Lead or Lag  PoleZ=0.95  ZeroZ=0.75  ICPrevOutput=0.0  ICPrevInput=0.0  DoSatur=off
      settings: SourceProductBaseCode=SL
  cfblk4 : Constant  Value=[-908917448.180678]  SampleTime=1
  cfblk2 : Outport
  wires:
  cfblk1/1 -> cfblk2/1
  cfblk4/1 -> cfblk3/1

== system sampleModel180/cfblk88 ==
  cfblk1 : Inport
  cfblk3 : Inport  Port=2
  cfblk2 : Outport
  wires:
  cfblk3/1 -> cfblk2/1

== system sampleModel180/cfblk89 ==
  cfblk1 : Inport
  cfblk3 : Product
  cfblk2 : Outport
  wires:
  cfblk1/1 -> cfblk3/1, cfblk3/2
  cfblk3/1 -> cfblk2/1

== system sampleModel180/cfblk90 ==
  cfblk1 : Inport
  cfblk4 : Inport  Port=2
  cfblk3 : Trigonometry
  cfblk2 : Outport
  wires:
  cfblk1/1 -> cfblk2/1
  cfblk4/1 -> cfblk3/1

== system sampleModel180/cfblk91 ==
  cfblk1 : Inport
  cfblk3 : Inport  Port=2
  cfblk4 : Inport  Port=3
  cfblk2 : Outport
  wires:
  cfblk1/1 -> cfblk2/1

== system sampleModel180/cfblk92 ==
  cfblk1 : Inport
  cfblk3 : Inport  Port=2
  cfblk2 : Outport
  cfblk4 : Outport  Port=2
  wires:
  cfblk1/1 -> cfblk4/1
  cfblk3/1 -> cfblk2/1

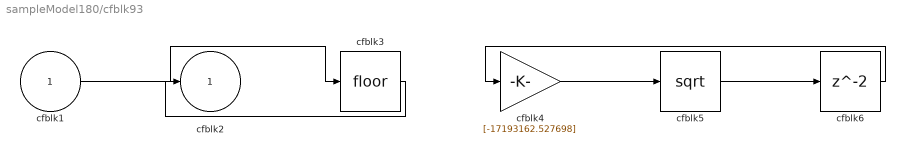
== system sampleModel180/cfblk93 ==
  cfblk1 : Inport
  cfblk3 : Rounding
  cfblk4 : Gain  Gain=[-17193162.527698]
  cfblk5 : Sqrt  SaturateOnIntegerOverflow=on
  cfblk6 : Delay  SampleTime=1
  cfblk2 : Outport
  wires:
  cfblk4/1 -> cfblk5/1
  cfblk1/1 -> cfblk3/1
  cfblk3/1 -> cfblk2/1
  cfblk5/1 -> cfblk6/1
  cfblk6/1 -> cfblk4/1

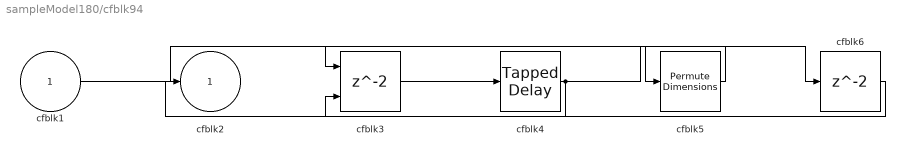
== system sampleModel180/cfblk94 ==
  cfblk1 : Inport
  cfblk3 : Delay  ShowEnablePort=on  SampleTime=1
      settings: InputPortMap=u0,e6
  cfblk4 : simulink/Discrete/Tapped Delay  vinit=0.0  samptime=-1  NumDelays=1  DelayOrder=Oldest  includeCurrent=off
  cfblk5 : PermuteDimensions
  cfblk6 : Delay  SampleTime=1
  cfblk2 : Outport
  wires:
  cfblk3/1 -> cfblk4/1
  cfblk1/1 -> cfblk5/1
  cfblk4/1 -> cfblk2/1, cfblk6/1
  cfblk5/1 -> cfblk3/1
  cfblk6/1 -> cfblk3/2

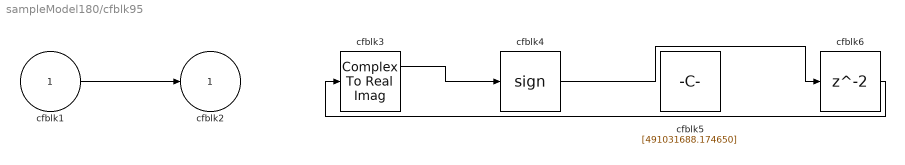
== system sampleModel180/cfblk95 ==
  cfblk1 : Inport
  cfblk3 : ComplexToRealImag
  cfblk4 : Signum
  cfblk5 : Constant  Value=[491031688.174650]  SampleTime=1
  cfblk6 : Delay  SampleTime=1
  cfblk2 : Outport
  wires:
  cfblk1/1 -> cfblk2/1
  cfblk3/1 -> cfblk4/1
  cfblk4/1 -> cfblk6/1
  cfblk6/1 -> cfblk3/1

== system sampleModel180/cfblk96 ==
  cfblk1 : Inport
  cfblk3 : Sin  TimeSource=Use external signal  SampleTime=0
  cfblk2 : Outport
  wires:
  cfblk1/1 -> cfblk3/1
  cfblk3/1 -> cfblk2/1
